simulink model "PI"  (R2018b)
settings: Solver=VariableStepAuto  StartTime=0.0  StopTime=4  RelTol=1e-3  EnableMultiTasking=on
values from neighbouring files (symbols this model uses):
  h = 0.1    [problema3_3.m]
  Ki_analog = wn^2    (= 25)    [problema3_3.m]
  Ki_discrete = Ki_analog * h/2    (= 1.25)    [problema3_3.m]
  Kp_analog = 2 * xi * wn - 1    (= 6)    [problema3_3.m]
  Kp_discrete = Kp_analog    (= 6)    [problema3_3.m]
undefined symbols (not defined in the file or in its folder): denG, numG
settings Model: Creator=IvoFrazão  LastModifiedBy=fredericovaz
settings OptimizationCC: LifeSpan=inf
settings DebuggingCC: SFUnexpectedBacktrackingDiag=warning  SFNoUnconditionalDefaultTransitionDiag=warning  SFExecutionAtInitializationDiag=none
settings SFSimCC: SimUseLocalCustomCode=off
settings RTWCC: RTWUseLocalCustomCode=off
settings CodeAppCC: StateflowObjectComments=on
settings GRTTargetCC: TargetLangStandard=C89/C90 (ANSI)  GeneratePreprocessorConditionals=Disable all
settings ConfigComp: CovMetricSettings=dw  CovHtmlReporting=on  CovSaveCumulativeToWorkspaceVar=on  CovSaveSingleToWorkspaceVar=on  CovExternalEMLEnable=off

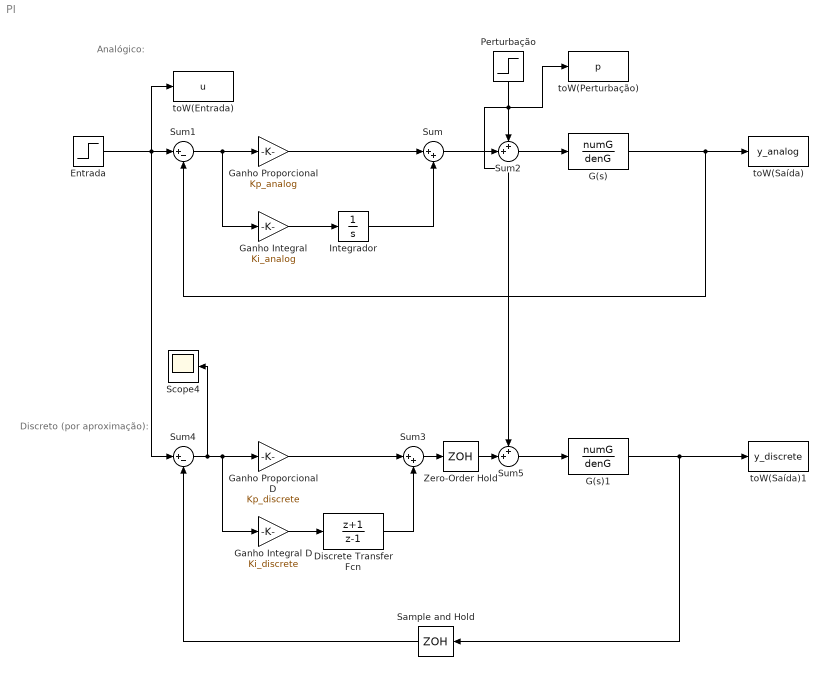
== system PI ==
  note: Analógico:
  note: Discreto (por aproximação):
  Discrete Transfer Fcn : DiscreteTransferFcn  Numerator=[1 1]  Denominator=[1 -1]  SampleTime=h
  Entrada : Step  Time=0.5  SampleTime=0
  G(s) : TransferFcn  Numerator=numG  Denominator=denG
  G(s)1 : TransferFcn  Numerator=numG  Denominator=denG
  Ganho Integral : Gain  Gain=Ki_analog
  Ganho Integral D : Gain  Gain=Ki_discrete
  Ganho Proporcional : Gain  Gain=Kp_analog
  Ganho Proporcional D : Gain  Gain=Kp_discrete
  Integrador : Integrator
  Perturbação : Step  Time=3  After=0.5  SampleTime=0
  Sample and Hold : ZeroOrderHold  SampleTime=h
  Scope4 : Scope
  Sum : Sum  Inputs=|++
  Sum1 : Sum  Inputs=|+-
  Sum2 : Sum  Inputs=++|
  Sum3 : Sum  Inputs=|++
  Sum4 : Sum  Inputs=|+-
  Sum5 : Sum  Inputs=++|
  Zero-Order Hold : ZeroOrderHold  SampleTime=h
  toW(Entrada) : ToWorkspace  VariableName=u  SaveFormat=Timeseries  SampleTime=-1
  toW(Perturbação) : ToWorkspace  VariableName=p  SaveFormat=Timeseries  SampleTime=-1
  toW(Saída) : ToWorkspace  VariableName=y_analog  SaveFormat=Timeseries  SampleTime=-1
  toW(Saída)1 : ToWorkspace  VariableName=y_discrete  SaveFormat=Timeseries  SampleTime=-1
  wires:
  Ganho Integral/1 -> Integrador/1
  Ganho Proporcional/1 -> Sum/1
  Integrador/1 -> Sum/2
  Sum1/1 -> Ganho Integral/1, Ganho Proporcional/1
  G(s)/1 -> toW(Saída)/1, Sum1/2
  Entrada/1 -> Sum4/1, toW(Entrada)/1, Sum1/1
  Sum/1 -> Sum2/2
  Sum2/1 -> G(s)/1
  Perturbação/1 -> toW(Perturbação)/1, Sum5/1, Sum2/1
  Ganho Proporcional D/1 -> Sum3/1
  Sum4/1 -> Scope4/1, Ganho Integral D/1, Ganho Proporcional D/1
  G(s)1/1 -> Sample and Hold/1, toW(Saída)1/1
  Sum5/1 -> G(s)1/1
  Ganho Integral D/1 -> Discrete Transfer Fcn/1
  Discrete Transfer Fcn/1 -> Sum3/2
  Sum3/1 -> Zero-Order Hold/1
  Zero-Order Hold/1 -> Sum5/2
  Sample and Hold/1 -> Sum4/2
